simulink model "Cruise"  (R2024a)
settings: Solver=ode23  StartTime=0.0  StopTime=10.0  RelTol=1e-3
libraries: slpidlib x1
settings Model: Creator=Envy 15  LastModifiedBy=Envy 15
settings SolverCC: ZeroCrossAlgorithm=Adaptive
settings DebuggingCC: IgnoredZcDiagnostic=none

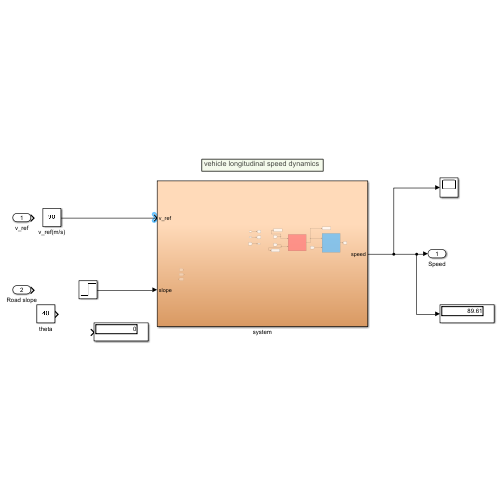
[thumbnail: Simulink's stored preview of the top-level diagram]
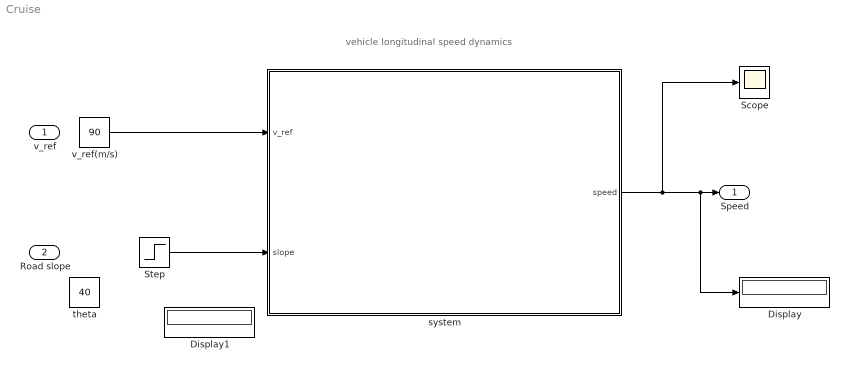
== system Cruise ==
  note: vehicle longitudinal speed dynamics
  v_ref : Inport
  Road slope : Inport  Port=2
  Display : Display
  Display1 : Display
  Scope : Scope
  Step : Step  Time=20  After=30  SampleTime=0  ZeroCross=off
  system : Subsystem
  theta : Constant  Value=40
  v_ref(m/s) : Constant  Value=90
  Speed : Outport
  wires:
  system/1(speed) -> Scope/1, Display/1, Speed/1
  v_ref(m/s)/1 -> system/1(v_ref)
  Step/1 -> system/2(slope)

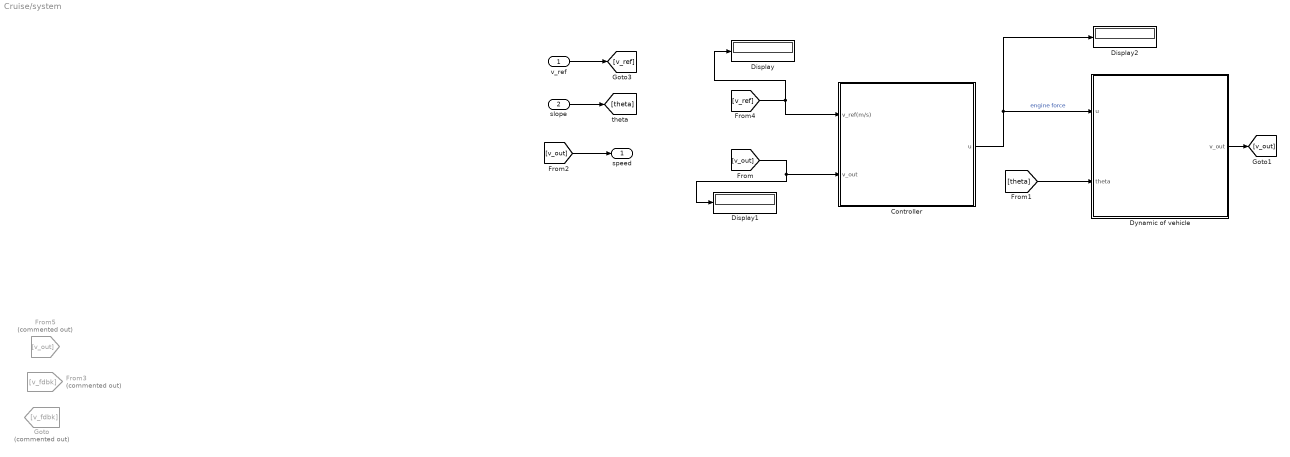
== system Cruise/system ==
  v_ref : Inport
  slope : Inport  Port=2
  Controller : Subsystem
  Display : Display
  Display1 : Display
  Display2 : Display
  Dynamic of vehicle : Subsystem
  From3 : From  Commented=on  GotoTag=v_fdbk
  From5 : From  Commented=on  GotoTag=v_out
  Goto : Goto  Commented=on  GotoTag=v_fdbk
  speed : Outport
  wires:
  v_ref/1 -> [v_ref]
  slope/1 -> [theta]
  [v_out] -> speed/1
  Dynamic of vehicle/1(v_out) -> [v_out]
  [v_out] -> Display1/1, Controller/2(v_out)
  [v_ref] -> Display/1, Controller/1(v_ref(m/s))
  Controller/1(u) -> Display2/1, Dynamic of vehicle/1(u)  "engine force"
  [theta] -> Dynamic of vehicle/2(theta)

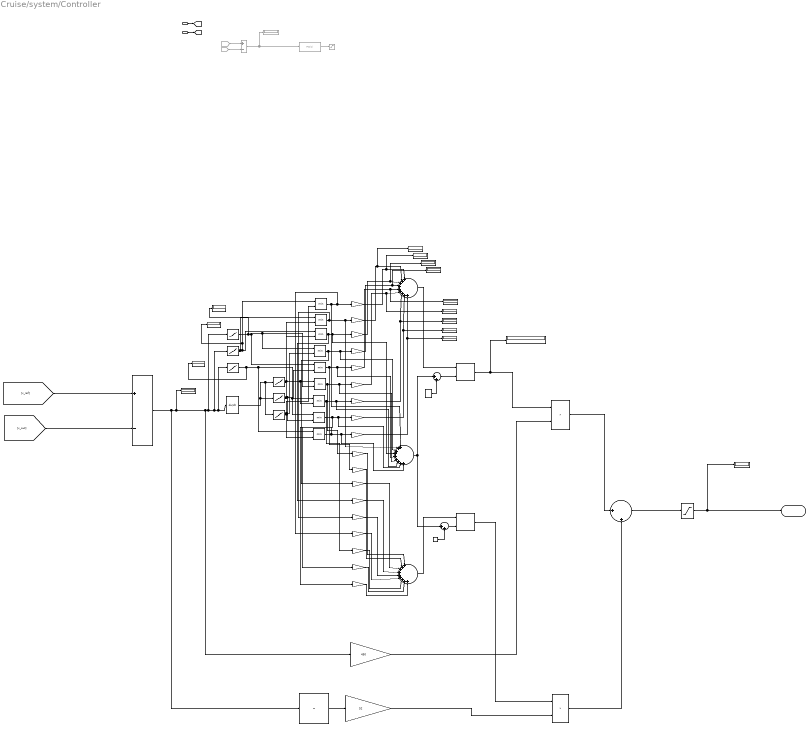
== system Cruise/system/Controller ==
  note: Math for the adaptive fuzzy PID:
      | Assume 3 sets for e : {Neg, Zero, Pos}
      | and 3 sets for de : {Neg, Zero, Pos} → total 9 rules .
      | Memberships:
      | $μde,j​(de),j∈{N1,Z1,P1}$
      | $μe,i​(e),i∈{N,Z,P}$
      | Rule firing strengths: (min blocks r₁…r₉)
      | $wij​=min(μe,i​(e),μde,j​(de))$
      | Local contributions of each rule:
      | $Kpij​=aPij​wij​$
      | $Kiij​=aIij​wij​$
      | Final adaptive gains:
      | $K_p(e,de) = \frac{\sum_{i,j} aP_{ij}\,w_{ij}}{\sum_{i,j} w_{ij}} % Adaptive fuzzy Ki K_i(e,de) = \frac{\sum_{i,j} aI_{ij}\,w_{ij}}{\sum_{i,j} w_{ij}}$
      | PID law with adaptive gains:
      | $u(t) = K_p(e,de)\,e(t) + K_i(e,de)\int e(t)\,dt$
  note: Notes for choosing gains:
      | For example:
      | When e≈0 but de<0, the speed is starting to drop; gain=1.5 boosts correction to stop drift early.
  note: Each min block computes the activation strength of one fuzzy rule.
      | For example: if e = –0.7 (strongly slow) and de = +0.4 (speed is improving), the rule is limited by the smaller truth value → min = 0.4.
      | This means the rule is only 40% active: ‘correct the speed, but not aggressively.’
  note: Breakpoints = [-10 −5 0] ,
      | Table data = [1 0 0] →
      | So: error −10 → μ=1 , error −5 → μ=0 , error 0 → μ=0 .
      |
      | The membership value says how much the current number “fits” the meaning of that fuzzy word.
      | A membership of 1 means “this number completely belongs to this category.”
      | A membership of 0 means “this number does NOT belong to this category at all.”
      | A value between 0 and 1 means “it belongs partly.”
      | A membership value can be any number between 0 and 1 , like 0.5.
      | For example for e=-7.5 , μ = 0.5 → “the error is moderately negative.”
  note: aI
  note: aP
  note: Weights
  note: strength of each fuzzy rule .
  note: fuzzy rules
  note: Memberships
  note: Memberships
  note: Normal PID
  note: What is ANTI-WINDUP? (Control Correction)
      | When the error is large AND the actuator is saturated:
      | The controller tries to fix error
      | It keeps INTEGRATING the error
      | But the actuator cannot do more
      | So the integrator keeps accumulating uselessly
      | This leads to: HUGE overshoot, VERY slow recovery, Oscillation,Unstable feeling
      | Anti-windup is: A correction mechanism that prevents the integral term from growing when the actuator is saturated.
  note: The goal for adding saturation:
      | In every real physical system:
      |
      | The engine cannot generate infinite force
      |
      | The throttle cannot go above 100%
      |
      | The motor cannot exceed maximum torque
      |
      | Brakes have limits
      |
      | Steering angle has limits
  v_ref(m/s) : Inport
  v_out : Inport  Port=2
  Constant : Constant  Value=1e-6
  Constant1 : Constant  Value=1e-6
  Derivative : Derivative
  Display : Display  Commented=on
  Display{1..15} (15 alike) : Display
  Divide : Product  Inputs=*/
  Divide1 : Product  Inputs=*/
  From : From  Commented=on  GotoTag=v_ref
  From1 : From  Commented=on  GotoTag=v_out
  Gain{,1,3,8,11,13..14,17} (8 alike) : Gain  Gain=0.5
  Gain{4,6,10,15} (4 alike) : Gain
  Gain{2,5,7,9,12,16} (6 alike) : Gain  Gain=1.5
  I_scale : Product
  Integrator : Integrator
  Ki0 : Gain  Gain=52
  Kp0 : Gain  Gain=450
  Minus : Sum  Commented=on  Inputs=+-
  Minus1 : Sum  Inputs=+-
  Negative : Lookup_n-D  NumberOfTableDimensions=1  BreakpointsForDimension1=[-10 -5 0]  Table="[1    0  0]"  InternalRulePriority=Speed  RndMeth=Simplest
  Negative1 : Lookup_n-D  NumberOfTableDimensions=1  BreakpointsForDimension1=[-10 -5 0]  Table="[1    0  0]"  InternalRulePriority=Speed  RndMeth=Simplest
  PID Controller : slpidlib/PID Controller  Commented=on  Controller=PID  Form=Parallel  TimeDomain=Continuous-time  UseExternalTs=off  SampleTime=-1  IntegratorMethod=Forward Euler  FilterMethod=Forward Euler  ControllerParametersSource=internal  P=300  I=53.7  UseKiTs=off  D=0  UseExternalDerivativeSource=off  N=0  UseFilter=on  TunerSelectOption=Transfer Function Based (PID Tuner App)  InitialConditionSource=internal  InitialConditionForIntegrator=0  InitialConditionForFilter=0  DifferentiatorICPrevScaledInput=0  ExternalReset=none  TrackingMode=off  Kt=1  LimitOutput=off  SatLimitsSource=internal  UpperSaturationLimit=inf  LowerSaturationLimit=-inf  LinearizeAsGain=on  AntiWindupMode=none  Kb=1  LimitIntegrator=off  UpperIntegratorSaturationLimit=inf  LowerIntegratorSaturationLimit=-inf  POutMin=[]  POutMax=[]  IOutMin=[]  IOutMax=[]  DOutMin=[]  DOutMax=[]  NOutMin=[]  NOutMax=[]  SumOutMin=[]  SumOutMax=[]  SaturationOutMin=[]  SaturationOutMax=[]  PParamMin=[]  PParamMax=[]  IParamMin=[]  IParamMax=[]  DParamMin=[]  DParamMax=[]  NParamMin=[]  NParamMax=[]  KbParamMin=[]  KbParamMax=[]  KtParamMin=[]  KtParamMax=[]  KbOutMin=[]  KbOutMax=[]  KtOutMin=[]  KtOutMax=[]  IntegratorOutMin=[]  IntegratorOutMax=[]  FilterOutMin=[]  FilterOutMax=[]  SumI1OutMin=[]  SumI1OutMax=[]  SumI2OutMin=[]  SumI2OutMax=[]  SumI3OutMin=[]  SumI3OutMax=[]  SumI4OutMin=[]  SumI4OutMax=[]  SumDOutMin=[]  SumDOutMax=[]  DifferentiatorOutMin=[]  DifferentiatorOutMax=[]  FilterDiffOutCoefMin=[]  FilterDiffOutCoefMax=[]  ReciprocalOutMin=[]  ReciprocalOutMax=[]  SumDenOutMin=[]  SumDenOutMax=[]  SumNumOutMin=[]  SumNumOutMax=[]  DivideOutMin=[]  DivideOutMax=[]  UdiffTsProdOutMin=[]  UdiffTsProdOutMax=[]  NTsProdOutMin=[]  NTsProdOutMax=[]  UintegralTsProdOutMin=[]  UintegralTsProdOutMax=[]  UngainTsProdOutMin=[]  UngainTsProdOutMax=[]  ClampingZeroOutDataTypeStr=Inherit: Inherit via back propagation  ClampingZeroOutMin=[]  ClampingZeroOutMax=[]  FilterDenConstantOutDataTypeStr=Inherit: Inherit via back propagation  FilterDenConstantOutMin=[]  FilterDenConstantOutMax=[]  PCopyOutDataTypeStr=Inherit: Inherit via back propagation  PCopyOutMin=[]  PCopyOutMax=[]  NCopyOutDataTypeStr=Inherit: Inherit via back propagation  NCopyOutMin=[]  NCopyOutMax=[]  IntegratorContinuousStateAttributes=''  IntegratorStateMustResolveToSignalObject=off  IntegratorRTWStateStorageClass=Auto  FilterContinuousStateAttributes=''  FilterStateMustResolveToSignalObject=off  FilterRTWStateStorageClass=Auto  ParallelPVariant=InternalParameters  IdealPVariant=Disabled  IVariant=InternalParameters  DVariant=InternalParameters  IntegratorVariant=Continuous  SatVariant=Disabled  AWVariant=Passthrough  PCopyVariant=Disabled  TRVariant=Disabled  FdbkBlocksVariant=Forward  IdealPFdbkVariant=Disabled  SatFdbkVariant=Disabled  DerivativeFilterVariant=ContFilter  NVariant=InternalParameters  NCopyVariant=Disabled  FilterICVariant=InternalICsFilter  IntegratorICVariant=InternalICs  ExternalResetVariant=Disabled  TRSumVariant=Passthrough  SumFdbkVariant=Disabled  SumVariant=Sum_PID  TsampFilterVariant=InternalTs  TsampNgainVariant=Passthrough  TsampIntegralVariant=Disabled_SignalSpec  ExternalSaturationOutDataTypeStr=Inherit: Same as second input  DerivativeSourceVariant=ErrorSignal
  P_scale : Product
  Positive : Lookup_n-D  NumberOfTableDimensions=1  BreakpointsForDimension1="[0  5  10]"  Table="[0   0  1]"  InternalRulePriority=Speed  RndMeth=Simplest
  Positive1 : Lookup_n-D  NumberOfTableDimensions=1  BreakpointsForDimension1="[0  5  10]"  Table="[0   0  1]"  InternalRulePriority=Speed  RndMeth=Simplest
  Saturation : Saturate  Commented=on  UpperLimit=5000  LowerLimit=0
  Saturation1 : Saturate  UpperLimit=50000  LowerLimit=0  ZeroCross=off
  Sum : Sum  Inputs=|++
  Sum1 : Sum  Inputs=|++
  Sum2 : Sum  Inputs=|++
  SumI : Sum  Inputs=|+++++++++
  SumRules : Sum  Inputs=|+++++++++
  Sump : Sum  Inputs=|+++++++++
  Zero : Lookup_n-D  NumberOfTableDimensions=1  BreakpointsForDimension1=[-5 0 5]  Table="[0    1  0]"  InternalRulePriority=Speed  RndMeth=Simplest
  Zero1 : Lookup_n-D  NumberOfTableDimensions=1  BreakpointsForDimension1=[-5 0 5]  Table="[0    1  0]"  InternalRulePriority=Speed  RndMeth=Simplest
  r{1..9} (9 alike) : MinMax  Inputs=2
  u : Outport
  wires:
  v_ref(m/s)/1 -> [v_ref]
  From/1 -> Minus/1
  v_out/1 -> [v_out]
  From1/1 -> Minus/2
  Minus/1 -> PID Controller/1, Display/1  "error"
  PID Controller/1 -> Saturation/1
  Saturation1/1 -> u/1, Display1/1
  Minus1/1 -> Integrator/1, Display2/1, Kp0/1, Negative/1, Zero/1, Positive/1, Derivative/1  "error"
  [v_ref] -> Minus1/1
  [v_out] -> Minus1/2
  Kp0/1 -> P_scale/2
  Derivative/1 -> Positive1/1, Negative1/1, Zero1/1  "de"
  Negative1/1 -> r4/2, r7/2, r1/1
  Negative/1 -> Display13/1, r3/1, r1/2, r2/1
  Zero1/1 -> r8/2, r2/2, r5/2
  Positive1/1 -> r6/2, r3/2, r9/2
  Zero/1 -> r5/1, Display14/1, r6/1, r4/1
  Positive/1 -> Display15/1, r8/1, r7/1, r9/1
  r6/1 -> SumRules/1, Gain14/1, Gain/1
  r5/1 -> Gain13/1, SumRules/2, Gain1/1
  r4/1 -> Gain12/1, SumRules/4, Gain2/1
  r2/1 -> Gain10/1, SumRules/5, Gain4/1
  r1/1 -> Gain9/1, SumRules/6, Gain5/1
  r7/1 -> Gain15/1, SumRules/7, Gain6/1
  r8/1 -> Gain16/1, SumRules/8, Gain7/1
  r9/1 -> Gain17/1, SumRules/9, Gain8/1
  Gain/1 -> Display5/1, Sump/1
  Gain1/1 -> Display4/1, Sump/2
  Gain2/1 -> Display6/1, Sump/3
  Gain3/1 -> Display7/1, Sump/4
  Gain4/1 -> Display8/1, Sump/5
  Gain5/1 -> Display9/1, Sump/6
  Gain6/1 -> Sump/7, Display10/1
  Gain7/1 -> Sump/8, Display11/1
  Gain8/1 -> Display12/1, Sump/9
  r3/1 -> Gain11/1, SumRules/3, Gain3/1
  Sump/1 -> Divide/1
  SumRules/1 -> Sum2/1, Sum1/1
  Gain9/1 -> SumI/1
  Gain10/1 -> SumI/2
  Gain11/1 -> SumI/3
  Gain12/1 -> SumI/4
  Gain13/1 -> SumI/5
  Gain14/1 -> SumI/6
  Gain15/1 -> SumI/7
  Gain16/1 -> SumI/8
  Gain17/1 -> SumI/9
  SumI/1 -> Divide1/1
  Integrator/1 -> Ki0/1
  Ki0/1 -> I_scale/2
  I_scale/1 -> Sum/2
  P_scale/1 -> Sum/1
  Sum/1 -> Saturation1/1
  Constant/1 -> Sum1/2
  Sum1/1 -> Divide1/2
  Constant1/1 -> Sum2/2
  Sum2/1 -> Divide/2
  Divide1/1 -> I_scale/1
  Divide/1 -> Display3/1, P_scale/1  "alpha_p"

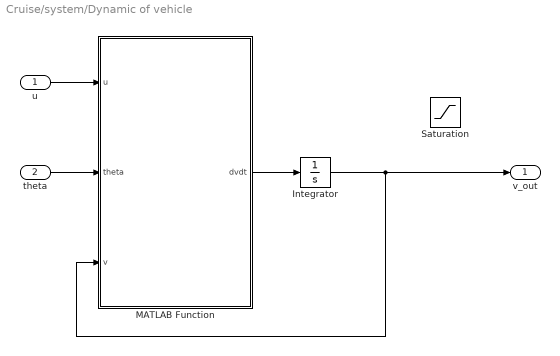
== system Cruise/system/Dynamic of vehicle ==
  u : Inport
  theta : Inport  Port=2
  Integrator : Integrator
  MATLAB Function : MATLAB Function  TreatAsAtomicUnit=on
  Saturation : Saturate  UpperLimit=120  ZeroCross=off
  v_out : Outport
  wires:
  u/1 -> MATLAB Function/1(u)
  theta/1 -> MATLAB Function/2(theta)
  MATLAB Function/1(dvdt) -> Integrator/1
  Integrator/1 -> MATLAB Function/3(v), v_out/1

== matlab function Cruise/system/Dynamic of vehicle/MATLAB Function ==
  data: u input; theta input; v input; dvdt output
function dvdt = vehicleDynamics(u, theta, v)
    % Parameters
    m = 1000;       % mass (kg)
    b = 50;         % drag coefficient (N*s/m)
    g = 9.81;       % gravity (m/s^2)

    % Vehicle dynamics
    dvdt = -(b/m)*v + (1/m)*u - g*sin(theta* pi/180);
end
